simulink model "elevation_control_2017"  (R2017b)
settings: Solver=VariableStepAuto  StartTime=0.0  StopTime=25.0  RelTol=1e-3
values from neighbouring files (symbols this model uses):
  deltaF_max = 3    [params.m]
undefined symbols (not defined in the file or in its folder): ddotE_F_Steady_den, ddotE_F_Steady_num
libraries: simulink x2
settings Model: Creator=bryankikuta  LastModifiedBy=bryankikuta
settings DataIOCC: ReturnWorkspaceOutputs=on
settings DebuggingCC: UnconnectedInputMsg=none  UnconnectedOutputMsg=none  UnconnectedLineMsg=none
settings ModelReferenceCC: EnableRefExpFcnMdlSchedulingChecks=off
settings SFSimCC: SimUseLocalCustomCode=on
settings RTWCC: Description=Generic Real-Time Target  RTWUseLocalCustomCode=on

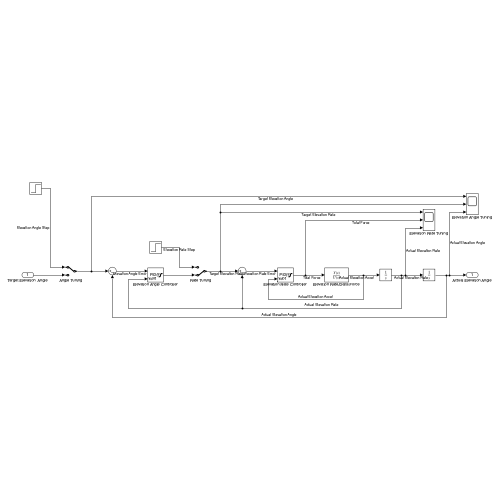
[thumbnail: Simulink's stored preview of the top-level diagram]
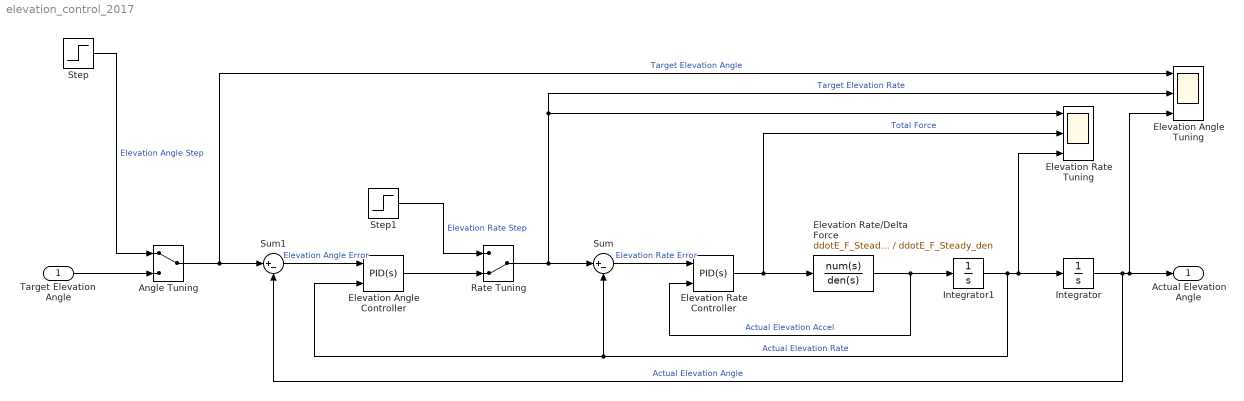
== system elevation_control_2017 ==
  Target Elevation  Angle : Inport
  Angle Tuning : ManualSwitch
  Elevation Angle Controller : simulink/Continuous/PID Controller  Controller=PID  Form=Parallel  TimeDomain=Continuous-time  SampleTime=-1  IntegratorMethod=Forward Euler  FilterMethod=Forward Euler  ControllerParametersSource=internal  P=3.5  I=0  D=1.9  N=1  UseFilter=on  TunerSelectOption=Transfer Function Based (PID Tuner App)  InitialConditionSource=internal  InitialConditionForIntegrator=0  InitialConditionForFilter=0  DifferentiatorICPrevScaledInput=0  ExternalReset=none  TrackingMode=off  Kt=1  LimitOutput=on  UpperSaturationLimit=pi/2  LowerSaturationLimit=-pi/2  LinearizeAsGain=off  AntiWindupMode=none  Kb=1  POutMin=[]  POutMax=[]  IOutMin=[]  IOutMax=[]  DOutMin=[]  DOutMax=[]  NOutMin=[]  NOutMax=[]  SumOutMin=[]  SumOutMax=[]  SaturationOutMin=[]  SaturationOutMax=[]  PParamMin=[]  PParamMax=[]  IParamMin=[]  IParamMax=[]  DParamMin=[]  DParamMax=[]  NParamMin=[]  NParamMax=[]  KbParamMin=[]  KbParamMax=[]  KtParamMin=[]  KtParamMax=[]  KbOutMin=[]  KbOutMax=[]  KtOutMin=[]  KtOutMax=[]  IntegratorOutMin=[]  IntegratorOutMax=[]  FilterOutMin=[]  FilterOutMax=[]  SumI1OutMin=[]  SumI1OutMax=[]  SumI2OutMin=[]  SumI2OutMax=[]  SumI3OutMin=[]  SumI3OutMax=[]  SumDOutMin=[]  SumDOutMax=[]  DifferentiatorOutMin=[]  DifferentiatorOutMax=[]  FilterDiffOutCoefMin=[]  FilterDiffOutCoefMax=[]  ReciprocalOutMin=[]  ReciprocalOutMax=[]  SumDenOutMin=[]  SumDenOutMax=[]  SumNumOutMin=[]  SumNumOutMax=[]  DivideOutMin=[]  DivideOutMax=[]  IntegratorContinuousStateAttributes=''  IntegratorStateMustResolveToSignalObject=off  IntegratorRTWStateStorageClass=Auto  FilterContinuousStateAttributes=''  FilterStateMustResolveToSignalObject=off  FilterRTWStateStorageClass=Auto  InitialConditionSetting=State (most efficient)
  Elevation Angle Tuning : Scope  NumInputPorts=3
  Elevation Rate Controller : simulink/Continuous/PID Controller  Controller=PID  Form=Parallel  TimeDomain=Continuous-time  SampleTime=-1  IntegratorMethod=Forward Euler  FilterMethod=Forward Euler  ControllerParametersSource=internal  P=6  I=1  D=3  N=20.0407888445835  UseFilter=on  TunerSelectOption=Transfer Function Based (PID Tuner App)  InitialConditionSource=internal  InitialConditionForIntegrator=0  InitialConditionForFilter=0  DifferentiatorICPrevScaledInput=0  ExternalReset=none  TrackingMode=off  Kt=1  LimitOutput=on  UpperSaturationLimit=deltaF_max  LowerSaturationLimit=-deltaF_max  LinearizeAsGain=off  AntiWindupMode=none  Kb=1  POutMin=[]  POutMax=[]  IOutMin=[]  IOutMax=[]  DOutMin=[]  DOutMax=[]  NOutMin=[]  NOutMax=[]  SumOutMin=[]  SumOutMax=[]  SaturationOutMin=[]  SaturationOutMax=[]  PParamMin=[]  PParamMax=[]  IParamMin=[]  IParamMax=[]  DParamMin=[]  DParamMax=[]  NParamMin=[]  NParamMax=[]  KbParamMin=[]  KbParamMax=[]  KtParamMin=[]  KtParamMax=[]  KbOutMin=[]  KbOutMax=[]  KtOutMin=[]  KtOutMax=[]  IntegratorOutMin=[]  IntegratorOutMax=[]  FilterOutMin=[]  FilterOutMax=[]  SumI1OutMin=[]  SumI1OutMax=[]  SumI2OutMin=[]  SumI2OutMax=[]  SumI3OutMin=[]  SumI3OutMax=[]  SumDOutMin=[]  SumDOutMax=[]  DifferentiatorOutMin=[]  DifferentiatorOutMax=[]  FilterDiffOutCoefMin=[]  FilterDiffOutCoefMax=[]  ReciprocalOutMin=[]  ReciprocalOutMax=[]  SumDenOutMin=[]  SumDenOutMax=[]  SumNumOutMin=[]  SumNumOutMax=[]  DivideOutMin=[]  DivideOutMax=[]  IntegratorContinuousStateAttributes=''  IntegratorStateMustResolveToSignalObject=off  IntegratorRTWStateStorageClass=Auto  FilterContinuousStateAttributes=''  FilterStateMustResolveToSignalObject=off  FilterRTWStateStorageClass=Auto  InitialConditionSetting=State (most efficient)
  Elevation Rate Tuning : Scope  NumInputPorts=3
  Elevation Rate/Delta Force : TransferFcn  Numerator=ddotE_F_Steady_num  Denominator=ddotE_F_Steady_den
  Integrator : Integrator
  Integrator1 : Integrator
  Rate Tuning : ManualSwitch  CurrentSetting=0
  Step : Step  After=24.5 * pi/180  SampleTime=0
  Step1 : Step  Time=0  After=pi/2  SampleTime=0
  Sum : Sum  Inputs=|+-
  Sum1 : Sum  Inputs=|+-
  Actual Elevation Angle : Outport
  wires:
  Step/1 -> Angle Tuning/1  "Elevation Angle Step"
  Sum/1 -> Elevation Rate Controller/1  "Elevation Rate Error"
  Integrator1/1 -> Elevation Rate Tuning/3, Integrator/1, Elevation Angle Controller/2, Sum/2  "Actual Elevation Rate"
  Elevation Rate Controller/1 -> Elevation Rate Tuning/2, Elevation Rate/Delta Force/1  "Total Force"
  Step1/1 -> Rate Tuning/1  "Elevation Rate Step"
  Rate Tuning/1 -> Elevation Angle Tuning/2, Elevation Rate Tuning/1, Sum/1  "Target Elevation Rate"
  Angle Tuning/1 -> Elevation Angle Tuning/1, Sum1/1  "Target Elevation Angle"
  Elevation Rate/Delta Force/1 -> Elevation Rate Controller/2, Integrator1/1  "Actual Elevation Accel"
  Integrator/1 -> Actual Elevation Angle/1, Elevation Angle Tuning/3, Sum1/2  "Actual Elevation Angle"
  Sum1/1 -> Elevation Angle Controller/1  "Elevation Angle Error"
  Target Elevation  Angle/1 -> Angle Tuning/2
  Elevation Angle Controller/1 -> Rate Tuning/2
